simulink model "chap4_4sim"  (Simulink 7.0)
settings: Solver=ode45  StartTime=0.0  StopTime=50  RelTol=1e-5
settings Model: Creator=hp  LastModifiedBy=eleliuj  ExtModeTrigMode=oneshot  ExtModeArmWhenConnect=off
settings DataIOCC: LimitDataPoints=off  SignalLoggingName=sigsOut
settings OptimizationCC: BooleanDataType=off
settings DebuggingCC: SaveWithParameterizedLinksMsg=none  SignalResolutionControl=TryResolveAllWithWarning  SolverPrmCheckMsg=none  MultiTaskDSMMsg=warning  MultiTaskCondExecSysMsg=none
settings HardwareCC: TargetUnknown=on
settings RTWCC: IncludeERTFirstTime=on
settings GRTTargetCC: TargetFcnLib=ansi_tfl_tmw.mat

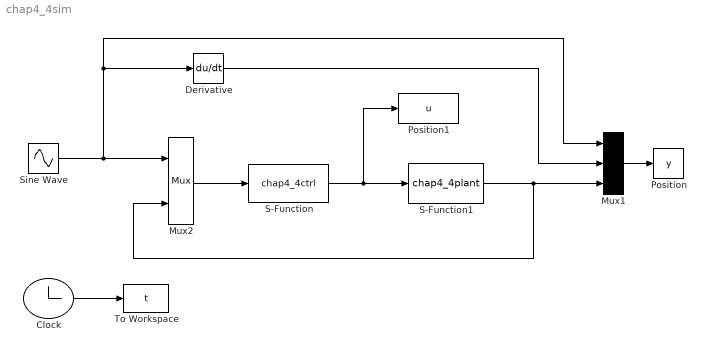
== system chap4_4sim ==
  Clock : Clock
      settings: Decimation=10
  Derivative : Derivative
  Mux1 : Mux  Inputs=3
  Mux2 : Mux  Inputs=2
  Position : ToWorkspace  VariableName=y  SampleTime=-1  SaveFormat=Array
  Position1 : ToWorkspace  VariableName=u  SampleTime=-1  SaveFormat=Array
  S-Function : S-Function  FunctionName=chap4_4ctrl
  S-Function1 : S-Function  FunctionName=chap4_4plant
  Sine Wave : Sin  SampleTime=0
  To Workspace : ToWorkspace  VariableName=t  SampleTime=-1  SaveFormat=Array
  wires:
  Mux1/1 -> Position/1
  S-Function1/1 -> Mux1/3, Mux2/2
  Clock/1 -> To Workspace/1
  Sine Wave/1 -> Mux2/1, Mux1/1, Derivative/1
  Mux2/1 -> S-Function/1
  S-Function/1 -> S-Function1/1, Position1/1
  Derivative/1 -> Mux1/2
